simulink model "ME322_Exercise_3_General_Case_Simulink"  (R2024b)
settings: Solver=VariableStepAuto  StartTime=0.0  StopTime=0.025  RelTol=1e-3
undefined symbols (not defined in the file or in its folder): x_i
settings Model: Creator=caidenbonney  LastModifiedBy=Caide

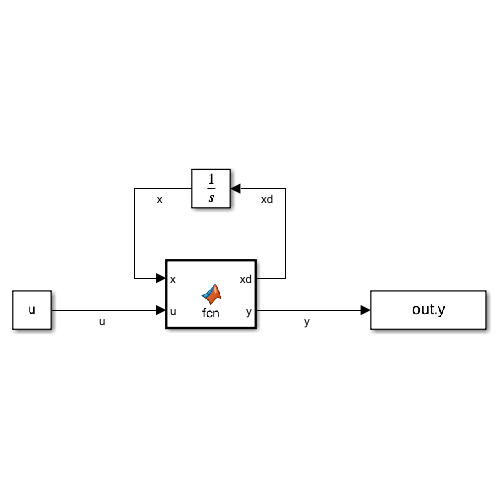
[thumbnail: Simulink's stored preview of the top-level diagram]
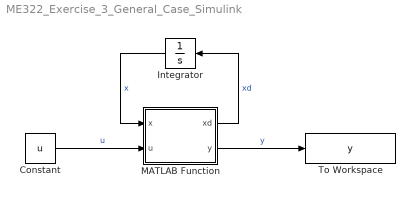
== system ME322_Exercise_3_General_Case_Simulink ==
  Constant : Constant  Value=u  VectorParams1D=off
  Integrator : Integrator  InitialCondition=x_i
  MATLAB Function : MATLAB Function  TreatAsAtomicUnit=on
  To Workspace : ToWorkspace  VariableName=y  SampleTime=-1
  wires:
  Constant/1 -> MATLAB Function/2(u)  "u"
  MATLAB Function/1(xd) -> Integrator/1  "xd"
  Integrator/1 -> MATLAB Function/1(x)  "x"
  MATLAB Function/2(y) -> To Workspace/1  "y"

== matlab function ME322_Exercise_3_General_Case_Simulink/MATLAB Function ==
  data: x input; xd output size=2; u input; y output size=5; p parameter
function [xd, y]= fcn(x, u, p)

% Separate state variables into individual elements
i_L = x(1);     % [A]
omega_J = x(2); % [rad/sec]

% Separate input variables into individual elements
v_m = u(1); % [V]
T_L = u(2); % [N*m]

% Required given constants units
% p.L_m % [mH]
L_m = p.L_m *10^-3;  % [mH] -> 10^-3 [H]
% p.R_m % [ohms]
% p.K_v % [V*sec/rad]

% p.J_m % [g/cm^2]
J_m = p.J_m *10^-7;  % [g*cm^2] -> 10^-7 [rad/sec^2)/N*m]^-1
% p.K_t % [N*m/A]
% p.b_m % [N*m/sec]

% State Equations
id_L = (1/(L_m))*(v_m - p.R_m*i_L - p.K_v*omega_J); % <-- State eq. f_1
    % the expected units of the derivative of current with respect to
    % time is [A/sec]
        % (1/[H])    *    ([V] - [ohms]*[A] - [V*sec/rad]*[rad/sec])
        % (1/[V/(A/sec)])*([V] -  [V/A]*[A] - [V*sec/rad]*[rad/sec])
        % ([(A/sec)/V]  * ([V] - [V] - [V])
        % ([(A/sec)/V)*[V]
        % [A/sec]
omegad_J = (1/J_m)*(p.K_t*i_L - p.b_m*omega_J - T_L); % <-- State eq. f_2
    % the expected units of the derivative of speed with respect to
    % time is [rad/sec^2]
        % (1/([rad/sec^2)/N*m]^-1))*([N*m/A]*[A]-[N*m/sec]*[rad/sec]-[N*m])
        % ([rad/sec^2)/N*m])    *   ([N*m] - [N*m] - [N*m])
        % ([rad/sec^2)/N*m])*[N*m]
        % [rad/sec^2]

xd = [id_L       % <-- State f_1 [A/sec]
      omegad_J]; % <-- State f_2 [rad/sec^2]

% Output Equations
P_e = v_m*i_L;        % <-- Output eq. g_3 Unit Check [V]*[A] = [W]
P_L = T_L*omega_J;    % <-- Output eq. g_4 Unit Check [N*m]*[rad/sec] = [W]
efficiency = P_L/P_e; % <-- Output eq. g_5 Unit Check [w]/[W] = [-]

y = [i_L          % <-- Output g_1 [A]
     omega_J      % <-- Output g_2 [rad/sec]
     P_e          % <-- Output g_3 [W]
     P_L          % <-- Output g_4 [W]
     efficiency]; % <-- Output g_5 [-]
